simulink library "INT_EISGov_SelectTrqLim"  (R2016b)
settings: Solver=VariableStepAuto  StartTime=0.0  StopTime=10.0  RelTol=1e-3
settings Model: Creator=liutao  LastModifiedBy=liutao

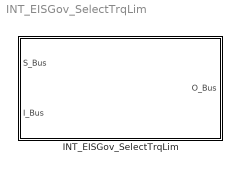
== system INT_EISGov_SelectTrqLim ==
  INT_EISGov_SelectTrqLim : Subsystem

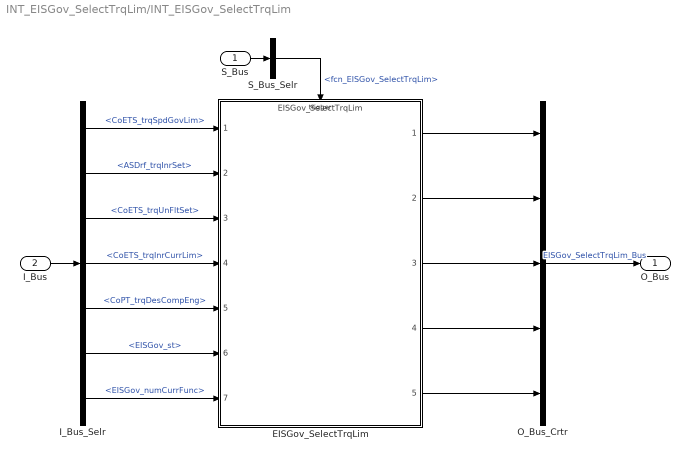
== system INT_EISGov_SelectTrqLim/INT_EISGov_SelectTrqLim ==
  S_Bus : Inport
  I_Bus : Inport  Port=2
  EISGov_SelectTrqLim : ModelReference  ModelNameDialog=EISGov_SelectTrqLim  SimulationMode=Normal  ModelReferenceVersion=1.26  TriggerPortName=function  TriggerPortTriggerType=function-call  TriggerPortStatesWhenEnabling=held
  I_Bus_Selr : BusSelector  OutputSignals=CoETS_trqSpdGovLim,ASDrf_trqInrSet,CoETS_trqUnFltSet,CoETS_trqInrCurrLim,CoPT_trqDesCompEng,EISGov_st,EISGov_numCurrFunc
  O_Bus_Crtr : BusCreator  Inputs=5
  S_Bus_Selr : BusSelector  OutputSignals=fcn_EISGov_SelectTrqLim
  O_Bus : Outport
  wires:
  S_Bus_Selr/1 -> EISGov_SelectTrqLim/Trigger  "<fcn_EISGov_SelectTrqLim>"
  S_Bus/1 -> S_Bus_Selr/1
  I_Bus/1 -> I_Bus_Selr/1
  I_Bus_Selr/1 -> EISGov_SelectTrqLim/1  "<CoETS_trqSpdGovLim>"
  I_Bus_Selr/2 -> EISGov_SelectTrqLim/2  "<ASDrf_trqInrSet>"
  I_Bus_Selr/3 -> EISGov_SelectTrqLim/3  "<CoETS_trqUnFltSet>"
  I_Bus_Selr/4 -> EISGov_SelectTrqLim/4  "<CoETS_trqInrCurrLim>"
  I_Bus_Selr/5 -> EISGov_SelectTrqLim/5  "<CoPT_trqDesCompEng>"
  I_Bus_Selr/6 -> EISGov_SelectTrqLim/6  "<EISGov_st>"
  I_Bus_Selr/7 -> EISGov_SelectTrqLim/7  "<EISGov_numCurrFunc>"
  O_Bus_Crtr/1 -> O_Bus/1  "EISGov_SelectTrqLim_Bus"
  EISGov_SelectTrqLim/1 -> O_Bus_Crtr/1
  EISGov_SelectTrqLim/2 -> O_Bus_Crtr/2
  EISGov_SelectTrqLim/3 -> O_Bus_Crtr/3
  EISGov_SelectTrqLim/4 -> O_Bus_Crtr/4
  EISGov_SelectTrqLim/5 -> O_Bus_Crtr/5
